simulink model "DAVID_JE_CSE_3_SIMULINK"  (R2024a)
settings: Solver=VariableStepAuto  StartTime=0.0  StopTime=20  RelTol=1e-3
values from neighbouring files (symbols this model uses):
  H_den = [M B k]    [DAVID_JE_CSE_3.m]
  H_num = [1]    [DAVID_JE_CSE_3.m]
settings Model: Creator=PC  LastModifiedBy=PC

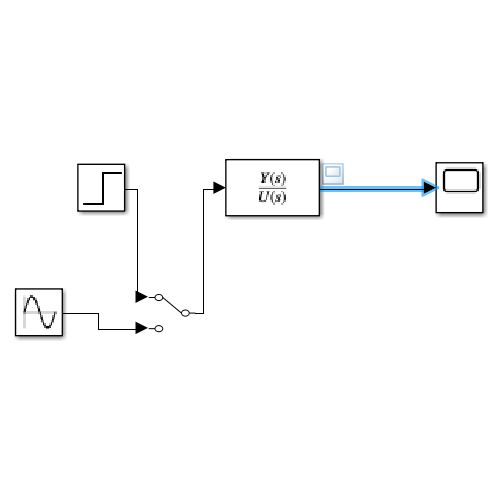
[thumbnail: Simulink's stored preview of the top-level diagram]
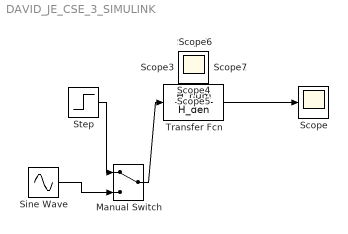
== system DAVID_JE_CSE_3_SIMULINK ==
  Manual Switch : ManualSwitch
  Scope{,1..7} (8 alike) : Scope
  Sine Wave : Sin  SampleTime=0
  Step : Step  Time=0  Before=0.1  SampleTime=0
  Transfer Fcn : TransferFcn  Numerator=H_num  Denominator=H_den
  wires:
  Step/1 -> Manual Switch/1
  Transfer Fcn/1 -> Scope/1
  Sine Wave/1 -> Manual Switch/2
  Manual Switch/1 -> Transfer Fcn/1
